simulink subsystem "PWMToForce"  (R2025b)
settings: Solver=VariableStepAuto  StartTime=0.0  StopTime=10.0  RelTol=1e-3
undefined symbols (not defined in the file or in its folder): dt_data, dt_sim
settings Model: Creator=koryh  LastModifiedBy=koryh

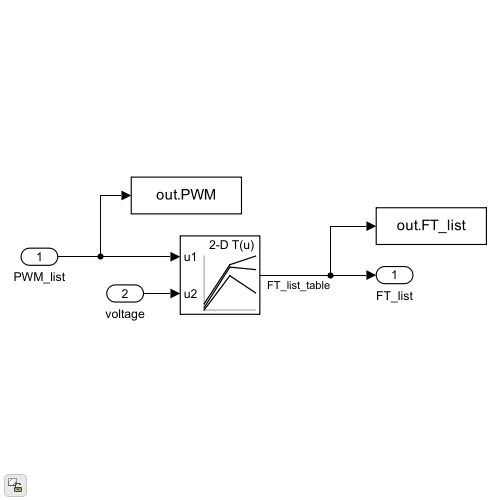
[thumbnail: Simulink's stored preview of the top-level diagram]
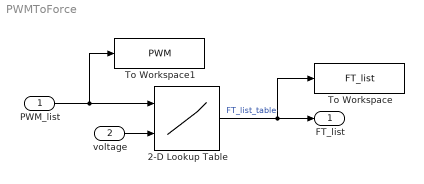
== system PWMToForce ==
  PWM_list : Inport  SampleTime=dt_sim
  voltage : Inport  Port=2
  2-D Lookup Table : Lookup_n-D  BreakpointsForDimension1=[1100;1104;1108;1112;1116;1120;1124;1128;1132;1136;1140;1144;1148;1152;1156;1160;1164;1168;1172;1176;1180;1184;1188;1192;1196;1200;1204;1208;1212;1216;1220;1224;1228;1232;1236;1240;1244;1248;1252;1256;1260;1264;1268;1272;1276;1280;1284;1288;1292;1296;1300;1304;1308;1312;1316;1320;1324;1328;1332;1336;1340;1344;1348;1352;1356;1360;1364;1368;1372;1376;1380;1384;1388;1392;1396;1400;1404;1408;1412;1416;1420;1424;1428;1432;1436;1440;1444;1448;1452;1456;1460;1464;1468;1472;1476;1480;1484;1488;1492;1496;1500;1504;1508;1512;1516;1520;1524;1528;1532;1536;1540;1544;1548;1552;1556;1560;1564;1568;1572;1576;1580;1584;1588;1592;1596;1600;1604;1608;1612;1616;1620;1624;1628;1632;1636;1640;1644;1648;1652;1656;1660;1664;1668;1672;1676;1680;1684;1688;1692;1696;1700;1704;1708;1712;1716;1720;1724;1728;1732;1736;1740;1744;1748;1752;1756;1760;1764;1768;1772;1776;1780;1784;1788;1792;1796;1800;1804;1808;1812;1816;1820;1824;1828;1832;1836;1840;1844;1848;1852;1856;1860;1864;1868;1872;1876;1880;1884;1888;1892;1896;1900]  BreakpointsForDimension2=[10;12;14;16;18;20]  Table=[-22.656600000000001 -28.485700000000001 -34.500300000000003 -39.921561779999998 -45.031300000000002 -49.399500000000003;-22.604700000000001 -28.611799999999999 -34.307499999999997 -39.736156049999998 -44.586399999999998 -48.635599999999997;-22.515699999999999 -28.389299999999999 -34.262999999999998 -39.469171799999998 -44.4529 -48.279699999999998;-22.382200000000001 -27.766400000000001 -33.862499999999997 -38.890705920000002 -43.918900000000001 -47.523200000000003;-21.803699999999999 -27.321400000000001 -33.372999999999998 -38.267742669999997 -43.340400000000002 -47.033700000000003;-21.403199999999998 -27.0989 -32.928100000000001 -37.956261050000002 -42.673000000000002 -46.5443;-21.225200000000001 -26.698399999999999 -32.305100000000003 -37.511287289999999 -42.628500000000003 -45.910800000000002;-20.913799999999998 -26.209 -31.860099999999999 -37.288800420000001 -40.893099999999997 -44.8979;-20.691299999999998 -25.497 -31.281700000000001 -36.799329290000003 -41.026600000000002 -43.785400000000003;-20.157299999999999 -25.452500000000001 -30.792200000000001 -36.443350289999998 -40.270099999999999 -43.207000000000001;-20.023800000000001 -25.140999999999998 -30.3917 -35.864884410000002 -39.602699999999999 -42.673000000000002;-19.489899999999999 -24.473600000000001 -29.991199999999999 -35.197423780000001 -39.157699999999998 -41.471600000000002;-19.1784 -23.939599999999999 -29.4573 -34.529963160000001 -38.401200000000003 -40.804099999999998;-18.9114 -23.8506 -28.834299999999999 -33.86250253 -37.8673 -40.403599999999997;-18.555399999999999 -23.4056 -28.3003 -33.328534019999999 -37.377800000000001 -39.424700000000001;-18.0214 -22.960599999999999 -27.944400000000002 -32.483083899999997 -36.443399999999997 -38.801699999999997;-17.7545 -22.604700000000001 -27.276900000000001 -31.904618020000001 -36.131900000000002 -38.134300000000003;-17.576499999999999 -22.115200000000002 -27.0989 -31.415146889999999 -34.885899999999999 -37.377800000000001;-17.220500000000001 -21.848199999999999 -26.386900000000001 -30.480702010000002 -34.752499999999998 -36.398899999999998;-16.82 -21.403199999999998 -25.942 -29.813241380000001 -33.595500000000001 -35.909399999999998;-16.508500000000002 -21.002800000000001 -25.452500000000001 -29.368267629999998 -32.928100000000001 -34.885899999999999;-16.196999999999999 -20.5578 -24.785 -28.834299130000002 -32.0381 -34.1295;-15.8856 -20.290800000000001 -24.429099999999998 -28.07784375 -31.3262 -32.928100000000001;-15.618600000000001 -19.712299999999999 -24.0731 -27.677367369999999 -30.347200000000001 -32.260599999999997;-15.262600000000001 -19.445399999999999 -23.6281 -27.187896250000001 -29.7242 -31.014700000000001;-15.0846 -19.089400000000001 -23.049600000000002 -26.564932989999999 -29.0123 -30.6587;-14.7286 -18.4664 -22.9161 -26.075461870000002 -28.255800000000001 -29.4573;-14.4171 -18.110399999999998 -22.159700000000001 -25.31900649 -27.899899999999999 -28.878799999999998;-14.1502 -17.710000000000001 -21.625699999999998 -25.00752486 -27.232399999999998 -28.166799999999999;-13.838699999999999 -17.443000000000001 -21.358699999999999 -24.60704849 -26.475899999999999 -27.232399999999998;-13.3492 -16.998000000000001 -20.7803 -24.073079979999999 -26.075500000000002 -26.831900000000001;-13.037699999999999 -16.330500000000001 -20.157299999999999 -23.36112198 -25.363499999999998 -26.209;-12.948700000000001 -16.196999999999999 -19.8903 -23.09413773 -24.785 -25.541499999999999;-12.6373 -15.7966 -19.489899999999999 -22.337682350000001 -24.2956 -24.963000000000001;-12.325799999999999 -15.3071 -18.7334 -21.937205970000001 -23.761600000000001 -24.5181;-11.969799999999999 -15.040100000000001 -18.555399999999999 -21.536729600000001 -23.1831 -23.895099999999999;-11.658300000000001 -14.6396 -17.843399999999999 -20.780274219999999 -22.738199999999999 -23.583600000000001;-11.4358 -14.4171 -17.3095 -20.424295220000001 -22.115200000000002 -22.6937;-11.168799999999999 -14.105700000000001 -16.8645 -19.845829340000002 -21.670200000000001 ...(+15050 chars)]  ExtrapMethod=Clip  UseLastTableValue=on  InternalRulePriority=Speed  RndMeth=Simplest
      settings: InputPortMap=u0,u1
  To Workspace : ToWorkspace  VariableName=FT_list  SaveFormat=Timeseries  SampleTime=dt_data
  To Workspace1 : ToWorkspace  VariableName=PWM  SaveFormat=Timeseries  SampleTime=dt_data
  FT_list : Outport
  wires:
  voltage/1 -> 2-D Lookup Table/2
  2-D Lookup Table/1 -> To Workspace/1, FT_list/1  "FT_list_table"
  PWM_list/1 -> 2-D Lookup Table/1, To Workspace1/1
